simulink model "UDP_example2"  (R2020b)
settings: Solver=FixedStepDiscrete  StartTime=0.0  StopTime=inf  FixedStep=0.001  RelTol=1e-3  EnableMultiTasking=on
libraries: eeGeneralControl x6, simulink x3, slrealtimeutilitieslib x1, sldrtlib x1, slrealtimeiplib x1, dspmtrx3 x1
settings Model: xpc_rtwmakecfg_data=_xpcetherlib__xpcether8255xlib__xpcetherGbElib__xpcnblib__xpciplib_  Creator=GreenRig  LastModifiedBy=danielh
settings DataIOCC: LimitDataPoints=on  ReturnWorkspaceOutputs=off
settings OptimizationCC: LifeSpan=inf
settings DebuggingCC: AllowSymbolicDim=off  PregeneratedLibrarySubsystemCodeDiagnostic=none  SFUnexpectedBacktrackingDiag=warning  SFNoUnconditionalDefaultTransitionDiag=warning  SFExecutionAtInitializationDiag=none  ArithmeticOperatorsInVariantConditions=warning
settings ModelReferenceCC: PropagateSignalLabelsOutOfModel=off
settings SFSimCC: SimUseLocalCustomCode=off  CustomCodeUndefinedFunction=UseInterfaceOnly
settings RTWCC: RTWUseLocalCustomCode=off
settings CodeAppCC: StateflowObjectComments=on
settings GRTTargetCC: TargetLangStandard=C89/C90 (ANSI)
settings ConfigComp: CovMetricSettings=dw  CovSaveCumulativeToWorkspaceVar=on  CovSaveSingleToWorkspaceVar=on  CovExternalEMLEnable=off  PLC_TargetIDE=indraworks  PLC_GenerateReport=off  PLC_LaunchReport=off
settings SimscapeCC: SimscapeNormalizeSystem=off
settings ConfigurationSet: Description=SimMechanics 2G

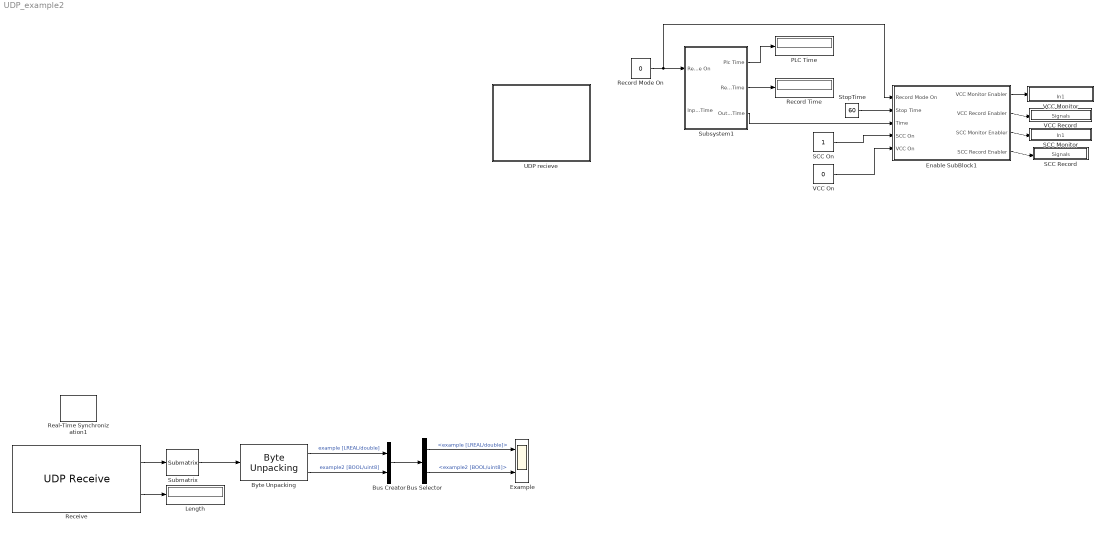
== system UDP_example2 ==
  Bus Creator : BusCreator  Inputs=2
  Bus Selector : BusSelector  OutputSignals=example [LREAL/double],example2 [BOOL/uint8]
  "Byte Unpacking " : slrealtimeutilitieslib/Byte Unpacking  MaskUnpackedDataTypes={'double','uint8'}  MaskUnpackedDataSizes={[1],[1]}  MaskAlignment=1
      settings: SourceProductBaseCode=XP
  Enable SubBlock1 : Subsystem
  Example : Scope  NumInputPorts=2
  Length : Display
  PLC Time : Display
      settings: Decimation=5
  Real-Time Synchronization1 : sldrtlib/Real-Time Synchronization  SampleTime=0.001  MaxMissedTicks=10000  ShowMissedTicks=off  YieldWhenWaiting=off
  "Receive " : slrealtimeiplib/UDP Receive  useHostTargetConn=on  ipAddress=10.10.10.15  localPort=1203  rcvWidth=20+8  rcvFmAny=off  fmAddress=192.168.1.1  rcvMulticast=off  multicastAddress=[]  sampleTime=0.001
      settings: SourceProductBaseCode=XP
  Record Mode On : Constant  Value=0
  Record Time : Display
      settings: Decimation=5
  SCC Monitor : Subsystem
  SCC On : Constant
  SCC Record : Subsystem
  StopTime : Constant  Value=60
  Submatrix : dspmtrx3/Submatrix  RowSpan=Range of rows  RowStartMode=Index  RowStartIndex=21  RowEndMode=Last  RowEndIndex=1  ColSpan=Range of columns  ColStartMode=First  ColStartIndex=1  ColEndMode=Last  ColEndIndex=1
  Subsystem1 : Subsystem
  UDP recieve : Subsystem
  VCC Monitor : Subsystem
  VCC On : Constant  Value=0
  VCC Record : Subsystem
  wires:
  StopTime/1 -> Enable SubBlock1/2(Stop Time)
  SCC On/1 -> Enable SubBlock1/4(SCC On)
  VCC On/1 -> Enable SubBlock1/5(VCC On)
  Subsystem1/2(Record Time) -> Record Time/1
  Subsystem1/1(Plc Time) -> PLC Time/1
  Subsystem1/3("Output Time ") -> Enable SubBlock1/3(Time)
  Record Mode On/1 -> Enable SubBlock1/1(Record Mode On), Subsystem1/1(Record Mode On)
  Enable SubBlock1/1(VCC Monitor Enabler) -> VCC Monitor/Action
  Enable SubBlock1/2(VCC Record Enabler) -> VCC Record/Action
  Enable SubBlock1/4(SCC Record Enabler) -> SCC Record/Action
  Enable SubBlock1/3(SCC Monitor Enabler) -> SCC Monitor/Action
  ? -> Subsystem1/2(Input Time), SCC Record/1(Signals), SCC Monitor/1(In1), VCC Record/1(Signals), VCC Monitor/1(In1)
  "Receive "/2 -> Length/1
  "Receive "/1 -> Submatrix/1
  Submatrix/1 -> "Byte Unpacking "/1
  "Byte Unpacking "/1 -> Bus Creator/1  "example [LREAL/double]"
  Bus Creator/1 -> Bus Selector/1
  Bus Selector/1 -> Example/1  "<example [LREAL/double]>"
  "Byte Unpacking "/2 -> Bus Creator/2  "example2 [BOOL/uint8]"
  Bus Selector/2 -> Example/2  "<example2 [BOOL/uint8]>"

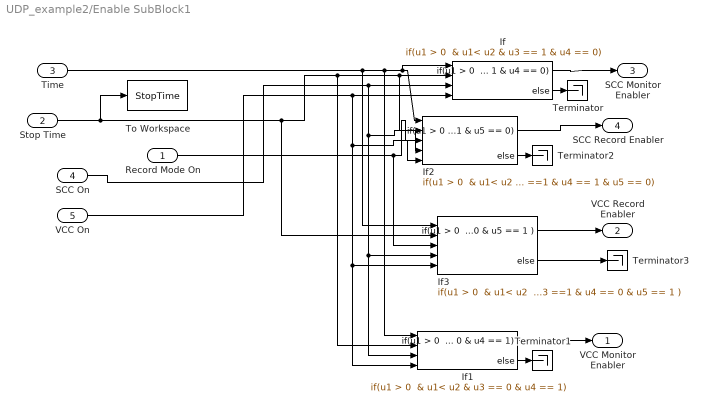
== system UDP_example2/Enable SubBlock1 ==
  Record Mode On : Inport
  Stop Time : Inport  Port=2
  Time : Inport  Port=3
  SCC On : Inport  Port=4
  VCC On : Inport  Port=5
  If : If  NumInputs=4  IfExpression="u1 > 0  & u1< u2 & u3 == 1 & u4 == 0"
  If1 : If  NumInputs=4  IfExpression="u1 > 0  & u1< u2 & u3 == 0 & u4 == 1"
  If2 : If  NumInputs=5  IfExpression="u1 > 0  & u1< u2  & u3 ==1 & u4 == 1 & u5 == 0"
  If3 : If  NumInputs=5  IfExpression="u1 > 0  & u1< u2  & u3 ==1 & u4 == 0 & u5 == 1"
  Terminator{,1..3} (4 alike) : Terminator
  To Workspace : ToWorkspace  VariableName=StopTime  SampleTime=-1
      settings: MaxDataPoints=1
  VCC Monitor Enabler : Outport  VectorParamsAs1DForOutWhenUnconnected=off
  VCC Record Enabler : Outport  Port=2  VectorParamsAs1DForOutWhenUnconnected=off
  SCC Monitor Enabler : Outport  Port=3  VectorParamsAs1DForOutWhenUnconnected=off
  SCC Record Enabler : Outport  Port=4  VectorParamsAs1DForOutWhenUnconnected=off
  wires:
  If/1 -> SCC Monitor Enabler/1
  If/2 -> Terminator/1
  Stop Time/1 -> To Workspace/1, If3/2, If1/2, If2/2, If/2
  Time/1 -> If3/1, If1/1, If2/1, If/1
  If1/1 -> VCC Monitor Enabler/1
  If1/2 -> Terminator1/1
  SCC On/1 -> If2/4, If3/4, If1/3, If/3
  VCC On/1 -> If2/5, If3/5, If1/4, If/4
  If2/1 -> SCC Record Enabler/1
  If2/2 -> Terminator2/1
  Record Mode On/1 -> If2/3, If3/3
  If3/1 -> VCC Record Enabler/1
  If3/2 -> Terminator3/1

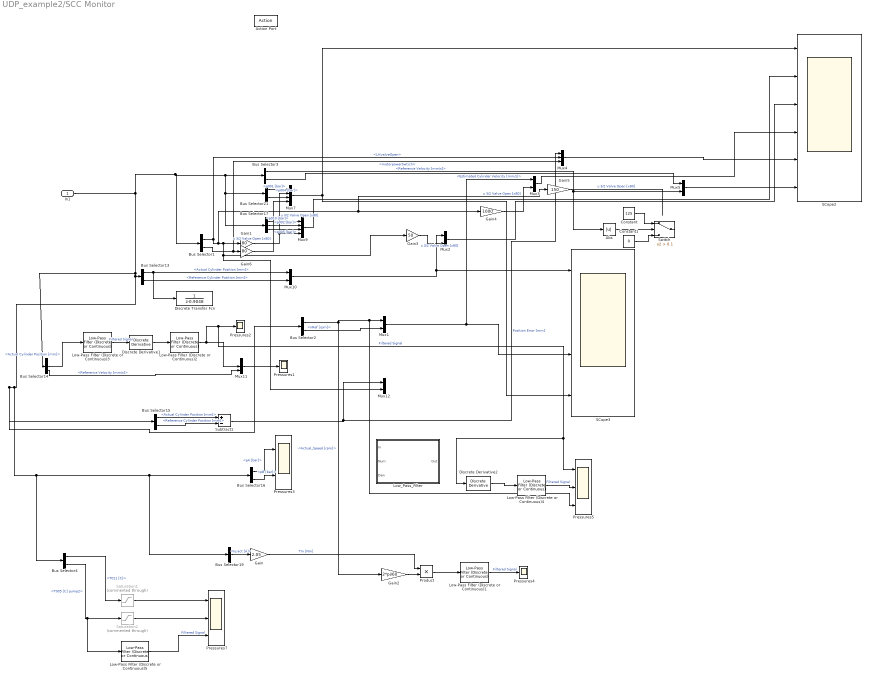
== system UDP_example2/SCC Monitor ==
  In1 : Inport
  Action Port : ActionPort  ActionPortLabel="if(u1 > 0  & u1< u2 & u3 == 1 & u4 == 0)"
  Abs : Abs
  Bus Selector1 : BusSelector  OutputSignals=LHvalveOpen,motorpowerSwtich
  Bus Selector13 : BusSelector  OutputSignals=Actual Cylinder Position [mm],Reference Cylinder Position [mm]
  Bus Selector14 : BusSelector  OutputSignals=Estimated Cylinder Velocity [mm/s],Actual Cylinder Position [mm],Reference Velocity [mm/s]
  Bus Selector15 : BusSelector  OutputSignals=Actual Cylinder Position [mm],Reference Cylinder Position [mm]
  Bus Selector16 : BusSelector  OutputSignals=pA [bar],pB [bar]
  Bus Selector17 : BusSelector  OutputSignals=p010 [bar],p002 [bar],p005 [bar]
  Bus Selector19 : BusSelector  OutputSignals=Iq act [A]
  Bus Selector2 : BusSelector  OutputSignals=Actual_Speed [rpm],nRef [rpm]
  Bus Selector21 : BusSelector  OutputSignals=p001 [bar],p004 [bar]
  Bus Selector3 : BusSelector  OutputSignals=Reference Velocity [mm/s],Estimated Cylinder Velocity [mm/s]
  Bus Selector4 : BusSelector  OutputSignals=T011 [C],T005 [C] pump2
  Constant : Constant  Value=125
  Constant1 : Constant  Value=0
  Discrete Transfer Fcn : DiscreteTransferFcn  Denominator=[1 -0.9048]
  Discrete Derivative1 : simulink/Discrete/Discrete Derivative  gainval=1.0  ICPrevScaledInput=0.0  OutMin=[]  OutMax=[]  OutDataType=fixdt(1, 16)  OutScaling=2^-10  DoSatur=off
  Discrete Derivative2 : simulink/Discrete/Discrete Derivative  gainval=1.0  ICPrevScaledInput=0.0  OutMin=[]  OutMax=[]  OutDataType=fixdt(1, 16)  OutScaling=2^-10  DoSatur=off
  Gain : Gain  Gain=2.05
  Gain1 : Gain  Gain=80
  Gain2 : Gain  Gain=2*pi/60
  Gain3 : Gain  Gain=50
  Gain4 : Gain  Gain=1000
  Gain5 : Gain  Gain=150
  Gain6 : Gain  Gain=80
  Low-Pass Filter (Discrete or Continuous)1 : eeGeneralControl/Low-Pass Filter (Discrete or Continuous)  K=1  T=0.05  B=inf  A=-inf  init_option=Inherited from block input  x0=0  Ts=-1
  Low-Pass Filter (Discrete or Continuous){2..5} (4 alike) : eeGeneralControl/Low-Pass Filter (Discrete or Continuous)  K=1  T=0.05  B=200  A=-200  init_option=Inherited from block input  x0=0  Ts=-1
  Low_Pass_Filter : Subsystem  TreatAsAtomicUnit=on
  Mux{1..3,5,10,12} (6 alike) : Mux  Inputs=2
  Mux11 : Mux  Inputs=3
  Mux4 : Mux  Inputs=3
  Mux7 : Mux
  Mux9 : Mux
  Pressures1 : Scope
  Pressures2 : Scope
  Pressures3 : Scope  NumInputPorts=2
  Pressures4 : Scope
  Pressures5 : Scope  NumInputPorts=3
  Pressures7 : Scope  NumInputPorts=3
  Product : Product
  SCope2 : Scope  NumInputPorts=6
  SCope3 : Scope  NumInputPorts=4
  Saturation1 : Saturate  Commented=through  UpperLimit=5  LowerLimit=-5
  Saturation2 : Saturate  Commented=through  UpperLimit=5  LowerLimit=-5
  Subtract1 : Sum  Inputs=+-
  Switch : Switch  Criteria=u2 > Threshold  Threshold=0.1
  wires:
  Bus Selector14/3 -> Mux11/3  "<Reference Velocity [mm/s]>"
  Gain1/1 -> Mux7/3, Mux9/4  "u 3/2 Valve Open [x80]"
  Gain/1 -> Product/1  "Tm [Nm]"
  Bus Selector1/1 -> Gain5/1, Gain4/1, Gain3/1, Mux12/2, Gain1/1, Mux4/2  "<LHvalveOpen>"
  Bus Selector16/1 -> Pressures3/1  "<pA [bar]>"
  Subtract1/1 -> Mux4/1, Mux12/1  "Position Error [mm]"
  Bus Selector17/2 -> Mux9/2  "<p002 [bar]>"
  Bus Selector16/2 -> Pressures3/2  "<pB [bar]>"
  Bus Selector13/2 -> Mux10/2  "<Reference Cylinder Position [mm]>"
  Mux9/1 -> SCope2/2
  Bus Selector17/1 -> Mux9/1  "<p010 [bar]>"
  Bus Selector13/1 -> Discrete Transfer Fcn/1, Mux10/1  "<Actual Cylinder Position [mm]>"
  Bus Selector21/2 -> Mux7/2  "<p004 [bar]>"
  Mux10/1 -> Mux2/1, SCope3/1
  Bus Selector15/1 -> Subtract1/1  "<Actual Cylinder Position [mm]>"
  Bus Selector15/2 -> Subtract1/2  "<Reference Cylinder Position [mm]>"
  Bus Selector21/1 -> Mux7/1  "<p001 [bar]>"
  Bus Selector14/2 -> Low-Pass Filter (Discrete or Continuous)3/1  "<Actual Cylinder Position [mm]>"
  Bus Selector19/1 -> Gain/1  "<Iq act [A]>"
  Bus Selector2/1 -> Gain2/1, Pressures5/3, Mux1/1  "<Actual_Speed [rpm]>"
  Bus Selector2/2 -> Mux1/2  "<nRef [rpm]>"
  Mux1/1 -> Mux3/1, SCope3/3
  Mux7/1 -> SCope3/4, SCope2/1
  Gain2/1 -> Product/2
  Product/1 -> Low-Pass Filter (Discrete or Continuous)1/1
  Low-Pass Filter (Discrete or Continuous)1/1 -> Pressures4/1  "Filtered Signal"
  Mux11/1 -> Pressures1/1
  Discrete Derivative1/1 -> Low-Pass Filter (Discrete or Continuous)2/1
  Low-Pass Filter (Discrete or Continuous)2/1 -> Discrete Derivative2/1, Pressures5/1, Pressures2/1, Mux11/2  "Filtered Signal"
  Bus Selector17/3 -> Mux9/3  "<p005 [bar]>"
  Gain3/1 -> Mux2/2  "u 3/2 Valve Open [x80]"
  Mux2/1 -> SCope2/3
  Mux3/1 -> SCope2/4
  Gain4/1 -> Mux3/2  "u 3/2 Valve Open [x80]"
  Mux4/1 -> SCope2/5
  Mux5/1 -> SCope2/6
  Gain5/1 -> ?  "u 3/2 Valve Open [x80]"
  In1/1 -> Bus Selector1/1, Bus Selector17/1, Bus Selector21/1, Bus Selector3/1, Bus Selector14/1, Bus Selector2/1, Bus Selector15/1, Bus Selector4/1, Bus Selector19/1, Bus Selector16/1, Bus Selector13/1
  Bus Selector3/1 -> Mux5/2, Abs/1  "<Reference Velocity [mm/s]>"
  Abs/1 -> Switch/2
  Constant/1 -> Switch/1
  Constant1/1 -> Switch/3
  Bus Selector1/2 -> Mux4/3, Gain6/1  "<motorpowerSwtich>"
  Gain6/1 -> Mux7/4  "u 3/2 Valve Open [x80]"
  Bus Selector3/2 -> Mux5/1  "<Estimated Cylinder Velocity [mm/s]>"
  Low-Pass Filter (Discrete or Continuous)3/1 -> Discrete Derivative1/1  "Filtered Signal"
  Discrete Derivative2/1 -> Low-Pass Filter (Discrete or Continuous)4/1
  Low-Pass Filter (Discrete or Continuous)4/1 -> Pressures5/2  "Filtered Signal"
  Bus Selector4/1 -> Saturation1/1  "<T011 [C]>"
  Bus Selector4/2 -> Low-Pass Filter (Discrete or Continuous)5/1, Saturation2/1  "<T005 [C] pump2>"
  Saturation2/1 -> Pressures7/2
  Saturation1/1 -> Pressures7/1
  Low-Pass Filter (Discrete or Continuous)5/1 -> Pressures7/3  "Filtered Signal"

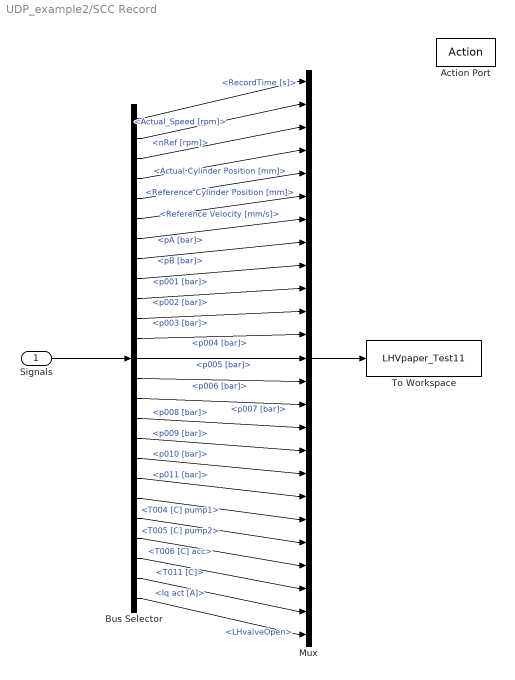
== system UDP_example2/SCC Record ==
  Signals : Inport
  Action Port : ActionPort  ActionPortLabel="if(u1 > 0  & u1< u2  & u3 ==1 & u4 == 1 & u5 == 0)"
  Bus Selector : BusSelector  OutputSignals=RecordTime [s],Actual_Speed [rpm],nRef [rpm],Actual Cylinder Position [mm],Reference Cylinder Position [mm],Reference Velocity [mm/s],pA [bar],pB [bar],p001 [bar],p002 [bar],p003 [bar],p004 [bar],p005 [bar],p006 [bar],p007 [bar],p008 [bar],p009 [bar],p010 [bar],p011 [bar],T004 [C] pump1,T005 [C] pump2,T006 [C] acc,T011 [C],Iq act [A],LHvalveOpen
  Mux : Mux  Inputs=25
  To Workspace : ToWorkspace  VariableName=LHVpaper_Test11  SampleTime=-1
      settings: Save2DSignal=2-D array (concatenate along first dimension)
  wires:
  Mux/1 -> To Workspace/1
  Bus Selector/1 -> Mux/1  "<RecordTime [s]>"
  Bus Selector/2 -> Mux/2  "<Actual_Speed [rpm]>"
  Bus Selector/3 -> Mux/3  "<nRef [rpm]>"
  Bus Selector/4 -> Mux/4  "<Actual Cylinder Position [mm]>"
  Bus Selector/5 -> Mux/5  "<Reference Cylinder Position [mm]>"
  Bus Selector/6 -> Mux/6  "<Reference Velocity [mm/s]>"
  Bus Selector/7 -> Mux/7  "<pA [bar]>"
  Bus Selector/8 -> Mux/8  "<pB [bar]>"
  Bus Selector/9 -> Mux/9  "<p001 [bar]>"
  Bus Selector/10 -> Mux/10  "<p002 [bar]>"
  Bus Selector/11 -> Mux/11  "<p003 [bar]>"
  Bus Selector/12 -> Mux/12  "<p004 [bar]>"
  Bus Selector/13 -> Mux/13  "<p005 [bar]>"
  Bus Selector/14 -> Mux/14  "<p006 [bar]>"
  Bus Selector/15 -> Mux/15  "<p007 [bar]>"
  Bus Selector/16 -> Mux/16  "<p008 [bar]>"
  Bus Selector/17 -> Mux/17  "<p009 [bar]>"
  Bus Selector/18 -> Mux/18  "<p010 [bar]>"
  Bus Selector/19 -> Mux/19  "<p011 [bar]>"
  Bus Selector/20 -> Mux/20  "<T004 [C] pump1>"
  Bus Selector/21 -> Mux/21  "<T005 [C] pump2>"
  Bus Selector/22 -> Mux/22  "<T006 [C] acc>"
  Bus Selector/23 -> Mux/23  "<T011 [C]>"
  Bus Selector/24 -> Mux/24  "<Iq act [A]>"
  Signals/1 -> Bus Selector/1
  Bus Selector/25 -> Mux/25  "<LHvalveOpen>"

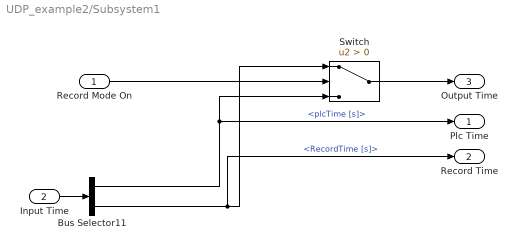
== system UDP_example2/Subsystem1 ==
  Record Mode On : Inport
  Input Time : Inport  Port=2
  Bus Selector11 : BusSelector  OutputSignals=plcTime [s],RecordTime [s]
  Switch : Switch  Criteria=u2 > Threshold
  Plc Time : Outport  VectorParamsAs1DForOutWhenUnconnected=off
  Record Time : Outport  Port=2  VectorParamsAs1DForOutWhenUnconnected=off
  "Output Time " : Outport  Port=3  VectorParamsAs1DForOutWhenUnconnected=off
  wires:
  Switch/1 -> "Output Time "/1
  Input Time/1 -> Bus Selector11/1
  Record Mode On/1 -> Switch/2
  Bus Selector11/1 -> Switch/3, Plc Time/1  "<plcTime [s]>"
  Bus Selector11/2 -> Switch/1, Record Time/1  "<RecordTime [s]>"

== system UDP_example2/UDP recieve ==
  wires:
  ? -> ?  "plcTime [s]"

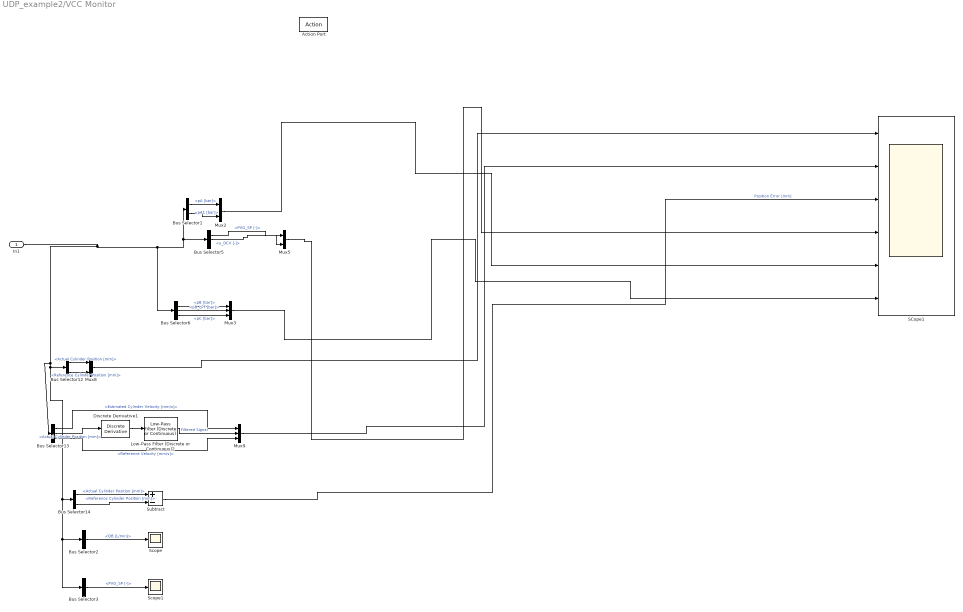
== system UDP_example2/VCC Monitor ==
  In1 : Inport
  Action Port : ActionPort  ActionPortLabel="if(u1 > 0  & u1< u2 & u3 == 0 & u4 == 1)"
  Bus Selector1 : BusSelector  OutputSignals=pA [bar],pA1 [bar]
  Bus Selector12 : BusSelector  OutputSignals=Actual Cylinder Position [mm],Reference Cylinder Position [mm]
  Bus Selector13 : BusSelector  OutputSignals=Estimated Cylinder Velocity [mm/s],Actual Cylinder Position [mm],Reference Velocity [mm/s]
  Bus Selector14 : BusSelector  OutputSignals=Actual Cylinder Position [mm],Reference Cylinder Position [mm]
  Bus Selector2 : BusSelector  OutputSignals=QB [L/min]
  Bus Selector3 : BusSelector  OutputSignals=PVG_SP [-]
  Bus Selector5 : BusSelector  OutputSignals=PVG_SP [-],u_DCV [-],u_PRV [-]
  Bus Selector6 : BusSelector  OutputSignals=pB [bar],pB_LPF [bar],pC [bar]
  Discrete Derivative1 : simulink/Discrete/Discrete Derivative  gainval=1.0  ICPrevScaledInput=0.0  OutMin=[]  OutMax=[]  OutDataType=fixdt(1, 16)  OutScaling=2^-10  DoSatur=off
  Low-Pass Filter (Discrete or Continuous)2 : eeGeneralControl/Low-Pass Filter (Discrete or Continuous)  K=1  T=0.01  B=150  A=-150  init_option=Inherited from block input  x0=0  Ts=-1
  Mux2 : Mux  Inputs=2
  Mux3 : Mux  Inputs=3
  Mux5 : Mux  Inputs=2
  Mux8 : Mux  Inputs=2
  Mux9 : Mux  Inputs=3
  SCope1 : Scope  NumInputPorts=6
  Scope : Scope
  Scope1 : Scope
  Subtract : Sum  Inputs=+-
  wires:
  Bus Selector1/2 -> Mux2/2  "<pA1 [bar]>"
  Bus Selector1/1 -> Mux2/1  "<pA [bar]>"
  Mux2/1 -> SCope1/5
  In1/1 -> Bus Selector13/1, Bus Selector3/1, Bus Selector2/1, Bus Selector14/1, Bus Selector12/1, Bus Selector5/1, Bus Selector1/1, Bus Selector6/1
  Bus Selector14/2 -> Subtract/2  "<Reference Cylinder Position [mm]>"
  Bus Selector13/2 -> Discrete Derivative1/1  "<Actual Cylinder Position [mm]>"
  Bus Selector5/2 -> Mux5/2  "<u_DCV [-]>"
  Bus Selector6/2 -> Mux3/2  "<pB_LPF [bar]>"
  Mux9/1 -> SCope1/2
  Mux5/1 -> SCope1/4
  Low-Pass Filter (Discrete or Continuous)2/1 -> Mux9/2  "Filtered Signal"
  Mux3/1 -> SCope1/6
  Discrete Derivative1/1 -> Low-Pass Filter (Discrete or Continuous)2/1
  Bus Selector12/2 -> Mux8/2  "<Reference Cylinder Position [mm]>"
  Bus Selector14/1 -> Subtract/1  "<Actual Cylinder Position [mm]>"
  Bus Selector6/1 -> Mux3/1  "<pB [bar]>"
  Subtract/1 -> SCope1/3  "Position Error [mm]"
  Bus Selector6/3 -> Mux3/3  "<pC [bar]>"
  Bus Selector5/1 -> Mux5/1  "<PVG_SP [-]>"
  Bus Selector13/3 -> Mux9/3  "<Reference Velocity [mm/s]>"
  Bus Selector2/1 -> Scope/1  "<QB [L/min]>"
  Bus Selector3/1 -> Scope1/1  "<PVG_SP [-]>"
  Bus Selector12/1 -> Mux8/1  "<Actual Cylinder Position [mm]>"
  Bus Selector13/1 -> Mux9/1  "<Estimated Cylinder Velocity [mm/s]>"
  Mux8/1 -> SCope1/1

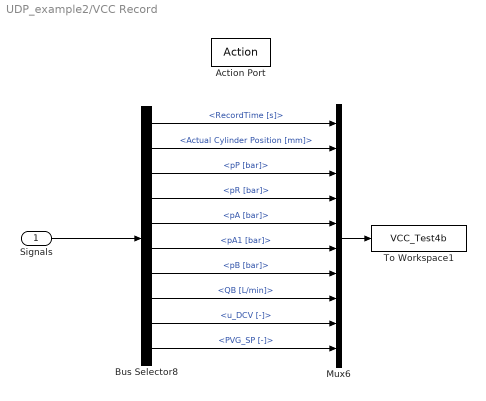
== system UDP_example2/VCC Record ==
  Signals : Inport
  Action Port : ActionPort  ActionPortLabel="if(u1 > 0  & u1< u2  & u3 ==1 & u4 == 0 & u5 == 1 )"
  Bus Selector8 : BusSelector  OutputSignals=RecordTime [s],Actual Cylinder Position [mm],pP [bar],pR [bar],pA [bar],pA1 [bar],pB [bar],QB [L/min],u_DCV [-],PVG_SP [-]
  Mux6 : Mux  Inputs=10
  To Workspace1 : ToWorkspace  VariableName=VCC_Test4b  SampleTime=-1
      settings: Save2DSignal=2-D array (concatenate along first dimension)
  wires:
  Signals/1 -> Bus Selector8/1
  Mux6/1 -> To Workspace1/1
  Bus Selector8/1 -> Mux6/1  "<RecordTime [s]>"
  Bus Selector8/2 -> Mux6/2  "<Actual Cylinder Position [mm]>"
  Bus Selector8/3 -> Mux6/3  "<pP [bar]>"
  Bus Selector8/4 -> Mux6/4  "<pR [bar]>"
  Bus Selector8/5 -> Mux6/5  "<pA [bar]>"
  Bus Selector8/6 -> Mux6/6  "<pA1 [bar]>"
  Bus Selector8/7 -> Mux6/7  "<pB [bar]>"
  Bus Selector8/8 -> Mux6/8  "<QB [L/min]>"
  Bus Selector8/9 -> Mux6/9  "<u_DCV [-]>"
  Bus Selector8/10 -> Mux6/10  "<PVG_SP [-]>"

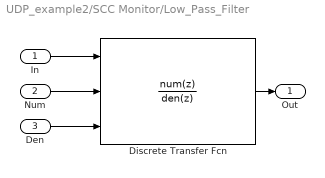
== system UDP_example2/SCC Monitor/Low_Pass_Filter ==
  In : Inport
  Num : Inport  Port=2
  Den : Inport  Port=3
  Discrete Transfer Fcn : DiscreteTransferFcn  NumeratorSource=Input port  DenominatorSource=Input port  a0EqualsOne=on
      settings: InputPortMap=u0,p1,p3
  Out : Outport  VectorParamsAs1DForOutWhenUnconnected=off
  wires:
  Num/1 -> Discrete Transfer Fcn/2
  Discrete Transfer Fcn/1 -> Out/1
  In/1 -> Discrete Transfer Fcn/1
  Den/1 -> Discrete Transfer Fcn/3
